simulink model "NRC_Template"  (R2025b)
settings: Solver=VariableStepAuto  StartTime=0.0  StopTime=10.0  RelTol=1e-3
undefined symbols (not defined in the file): ActivationSignal, ChargingWire, DataIN, DataLink, DataOUT, DCBus, DisplayLink, OutputWire, SwitchSignal
settings Model: Creator=jakeo  LastModifiedBy=nduka

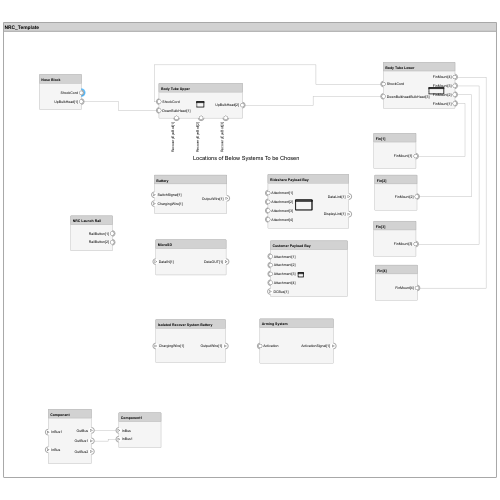
[thumbnail: Simulink's stored preview of the top-level diagram]
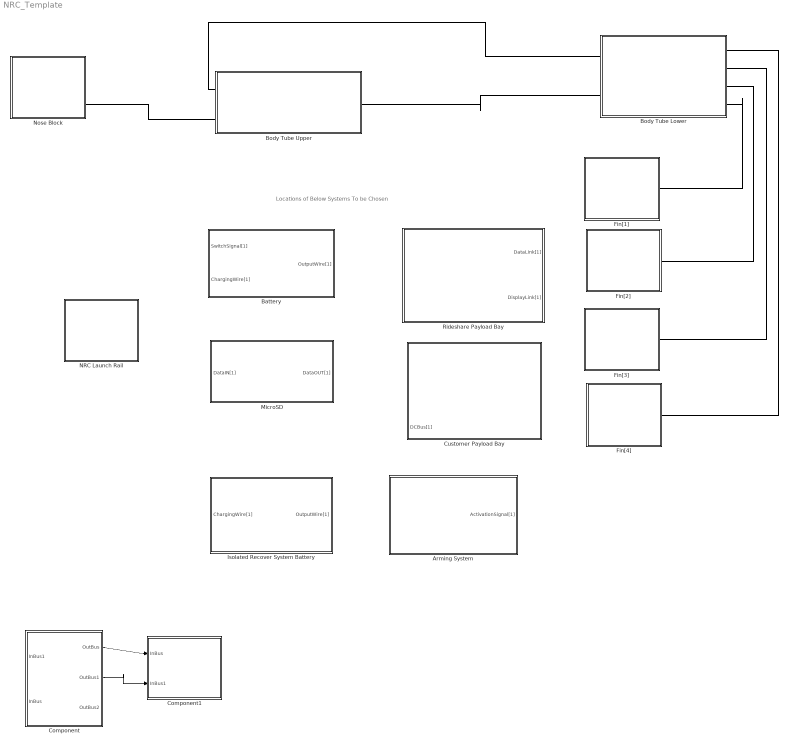
== system NRC_Template ==
  note: Locations of Below Systems To be Chosen
  Arming System : Subsystem
      settings: PortSchema="{\"entries\":[{\"content\":{\"headerSize\":26,\"margin\":15,\"minimumSpacing\":25,\"sides\":[{\"content\":{\"connectorIds\":[\"LConn1\"]},\"type\":\"ConnectorPlacement.EquallySpacedRectSide\",\"uuid\":\"6f4db608-f49c-4d1a-85cc-b66ec62c2f96\"},{\"content\":{\"connectorIds\":[\"Out1\"],\"side\":\"RIGHT\"},\"type\":\"ConnectorPlacement.EquallySpacedRectSide\",\"uuid\":\"3e275c67-1c5c-46cd-973f-75adcfca9e5d\"},{\"content\":{\"side\":\"TOP\"},\"type\":\"ConnectorPlacement.EquallySpacedRectSide\",\"uuid\":\"88fdcd36-c2bf-423f-a1bd-8e2b1c2ac438\"}]},\"type\":\"ConnectorPlacement.EquallySpacedConnector\",\"uuid\":\"596a3d77-8add-49e5-be48-e23e6a2b115a\"}],\"packageUris\":[\"http://schema.mathworks.com/mf0/Connector/R2020b\"],\"version\":\"1.0\"}"
  Battery : Subsystem
      settings: PortSchema="{\"entries\":[{\"content\":{\"headerSize\":26,\"margin\":15,\"minimumSpacing\":25,\"sides\":[{\"content\":{\"connectorIds\":[\"In1\",\"In2\"]},\"type\":\"ConnectorPlacement.EquallySpacedRectSide\",\"uuid\":\"03e957df-4bae-46ab-9d0d-48f80a496ac5\"},{\"content\":{\"connectorIds\":[\"Out1\"],\"side\":\"RIGHT\"},\"type\":\"ConnectorPlacement.EquallySpacedRectSide\",\"uuid\":\"d2433d43-ba0e-4345-8a8e-99b57dcef125\"},{\"content\":{\"side\":\"TOP\"},\"type\":\"ConnectorPlacement.EquallySpacedRectSide\",\"uuid\":\"84844adf-0e3d-439c-a28c-7cf27e8d243a\"}]},\"type\":\"ConnectorPlacement.EquallySpacedConnector\",\"uuid\":\"9b26577b-50b2-4983-8f3c-4df87f23ba49\"}],\"packageUris\":[\"http://schema.mathworks.com/mf0/Connector/R2020b\"],\"version\":\"1.0\"}"
  Body Tube Lower : Subsystem
      settings: PortSchema="{\"entries\":[{\"content\":{\"headerSize\":26,\"margin\":15,\"minimumSpacing\":25,\"sides\":[{\"content\":{\"connectorIds\":[\"LConn1\",\"LConn2\"]},\"type\":\"ConnectorPlacement.EquallySpacedRectSide\",\"uuid\":\"03e957df-4bae-46ab-9d0d-48f80a496ac5\"},{\"content\":{\"connectorIds\":[\"RConn1\",\"RConn2\",\"RConn3\",\"RConn4\"],\"side\":\"RIGHT\"},\"type\":\"ConnectorPlacement.EquallySpacedRectSide\",\"uuid\":\"d2433d43-ba0e-4345-8a8e-99b57dcef125\"},{\"content\":{\"side\":\"TOP\"},\"type\":\"ConnectorPlacement.EquallySpacedRectSide\",\"uuid\":\"84844adf-0e3d-439c-a28c-7cf27e8d243a\"}]},\"type\":\"ConnectorPlacement.EquallySpacedConnector\",\"uuid\":\"9b26577b-50b2-4983-8f3c-4df87f23ba49\"}],\"packageUris\":[\"http://schema.mathworks.com/mf0/Connector/R2020b\"],\"version\":\"1.0\"}"
  Body Tube Upper : Subsystem
      settings: PortSchema="{\"entries\":[{\"content\":{\"headerSize\":26,\"margin\":15,\"minimumSpacing\":25,\"sides\":[{\"content\":{\"connectorIds\":[\"LConn1\",\"LConn2\"]},\"type\":\"ConnectorPlacement.EquallySpacedRectSide\",\"uuid\":\"03e957df-4bae-46ab-9d0d-48f80a496ac5\"},{\"content\":{\"connectorIds\":[\"RConn1\"],\"side\":\"RIGHT\"},\"type\":\"ConnectorPlacement.EquallySpacedRectSide\",\"uuid\":\"d2433d43-ba0e-4345-8a8e-99b57dcef125\"},{\"content\":{\"side\":\"TOP\"},\"type\":\"ConnectorPlacement.EquallySpacedRectSide\",\"uuid\":\"84844adf-0e3d-439c-a28c-7cf27e8d243a\"},{\"content\":{\"connectorIds\":[\"RConn2\",\"RConn3\",\"RConn4\"],\"side\":\"BOTTOM\"},\"type\":\"ConnectorPlacement.EquallySpacedRectSide\",\"uuid\":\"7d79bddd-aaf5-48a9-85da-385393746c36\"}]},\"type\":\"ConnectorPlacement.EquallySpacedConnector\",\"uuid\":\"9b26577b-50b2-4983-8f3c-4df87f23ba49\"}],\"packageUris\":[\"http://schema.mathworks.com/mf0/Connector/R2020b\"],\"version\":\"1.0\"}"
  Component : Subsystem
      settings: PortSchema="{\"entries\":[{\"content\":{\"headerSize\":26,\"margin\":15,\"minimumSpacing\":25,\"sides\":[{\"content\":{\"connectorIds\":[\"In1\",\"In2\"]},\"type\":\"ConnectorPlacement.EquallySpacedRectSide\",\"uuid\":\"b214e6ac-d39e-436f-8c97-5d964e87c4ff\"},{\"content\":{\"connectorIds\":[\"Out1\",\"Out2\",\"Out3\"],\"side\":\"RIGHT\"},\"type\":\"ConnectorPlacement.EquallySpacedRectSide\",\"uuid\":\"c10b975c-0247-4c8e-aa32-d3b686cef9df\"},{\"content\":{\"side\":\"TOP\"},\"type\":\"ConnectorPlacement.EquallySpacedRectSide\",\"uuid\":\"84ce1942-2877-48a9-8a47-7e804e062fc7\"}]},\"type\":\"ConnectorPlacement.EquallySpacedConnector\",\"uuid\":\"8aac1783-a5cb-441e-81d2-9de359684d1e\"}],\"packageUris\":[\"http://schema.mathworks.com/mf0/Connector/R2020b\"],\"version\":\"1.0\"}"
  Component1 : Subsystem
      settings: PortSchema="{\"entries\":[{\"content\":{\"headerSize\":26,\"margin\":15,\"minimumSpacing\":25,\"sides\":[{\"content\":{\"connectorIds\":[\"In1\",\"In2\"]},\"type\":\"ConnectorPlacement.EquallySpacedRectSide\",\"uuid\":\"b214e6ac-d39e-436f-8c97-5d964e87c4ff\"},{\"content\":{\"side\":\"RIGHT\"},\"type\":\"ConnectorPlacement.EquallySpacedRectSide\",\"uuid\":\"c10b975c-0247-4c8e-aa32-d3b686cef9df\"},{\"content\":{\"side\":\"TOP\"},\"type\":\"ConnectorPlacement.EquallySpacedRectSide\",\"uuid\":\"84ce1942-2877-48a9-8a47-7e804e062fc7\"}]},\"type\":\"ConnectorPlacement.EquallySpacedConnector\",\"uuid\":\"8aac1783-a5cb-441e-81d2-9de359684d1e\"}],\"packageUris\":[\"http://schema.mathworks.com/mf0/Connector/R2020b\"],\"version\":\"1.0\"}"
  Customer Payload Bay : Subsystem
      settings: PortSchema="{\"entries\":[{\"content\":{\"headerSize\":26,\"margin\":15,\"minimumSpacing\":25,\"sides\":[{\"content\":{\"connectorIds\":[\"LConn1\",\"LConn2\",\"LConn3\",\"LConn4\",\"In1\"]},\"type\":\"ConnectorPlacement.EquallySpacedRectSide\",\"uuid\":\"03e957df-4bae-46ab-9d0d-48f80a496ac5\"},{\"content\":{\"side\":\"RIGHT\"},\"type\":\"ConnectorPlacement.EquallySpacedRectSide\",\"uuid\":\"d2433d43-ba0e-4345-8a8e-99b57dcef125\"},{\"content\":{\"side\":\"TOP\"},\"type\":\"ConnectorPlacement.EquallySpacedRectSide\",\"uuid\":\"84844adf-0e3d-439c-a28c-7cf27e8d243a\"}]},\"type\":\"ConnectorPlacement.EquallySpacedConnector\",\"uuid\":\"9b26577b-50b2-4983-8f3c-4df87f23ba49\"}],\"packageUris\":[\"http://schema.mathworks.com/mf0/Connector/R2020b\"],\"version\":\"1.0\"}"
  Fin[1] : Subsystem
      settings: PortSchema="{\"entries\":[{\"content\":{\"headerSize\":26,\"margin\":15,\"minimumSpacing\":25,\"sides\":[{\"content\":{},\"type\":\"ConnectorPlacement.EquallySpacedRectSide\",\"uuid\":\"03e957df-4bae-46ab-9d0d-48f80a496ac5\"},{\"content\":{\"connectorIds\":[\"LConn1\"],\"side\":\"RIGHT\"},\"type\":\"ConnectorPlacement.EquallySpacedRectSide\",\"uuid\":\"d2433d43-ba0e-4345-8a8e-99b57dcef125\"},{\"content\":{\"side\":\"TOP\"},\"type\":\"ConnectorPlacement.EquallySpacedRectSide\",\"uuid\":\"84844adf-0e3d-439c-a28c-7cf27e8d243a\"}]},\"type\":\"ConnectorPlacement.EquallySpacedConnector\",\"uuid\":\"9b26577b-50b2-4983-8f3c-4df87f23ba49\"}],\"packageUris\":[\"http://schema.mathworks.com/mf0/Connector/R2020b\"],\"version\":\"1.0\"}"
  Fin[2] : Subsystem
      settings: PortSchema="{\"entries\":[{\"content\":{\"headerSize\":26,\"margin\":15,\"minimumSpacing\":25,\"sides\":[{\"content\":{},\"type\":\"ConnectorPlacement.EquallySpacedRectSide\",\"uuid\":\"03e957df-4bae-46ab-9d0d-48f80a496ac5\"},{\"content\":{\"connectorIds\":[\"LConn1\"],\"side\":\"RIGHT\"},\"type\":\"ConnectorPlacement.EquallySpacedRectSide\",\"uuid\":\"d2433d43-ba0e-4345-8a8e-99b57dcef125\"},{\"content\":{\"side\":\"TOP\"},\"type\":\"ConnectorPlacement.EquallySpacedRectSide\",\"uuid\":\"84844adf-0e3d-439c-a28c-7cf27e8d243a\"}]},\"type\":\"ConnectorPlacement.EquallySpacedConnector\",\"uuid\":\"9b26577b-50b2-4983-8f3c-4df87f23ba49\"}],\"packageUris\":[\"http://schema.mathworks.com/mf0/Connector/R2020b\"],\"version\":\"1.0\"}"
  Fin[3] : Subsystem
      settings: PortSchema="{\"entries\":[{\"content\":{\"headerSize\":26,\"margin\":15,\"minimumSpacing\":25,\"sides\":[{\"content\":{},\"type\":\"ConnectorPlacement.EquallySpacedRectSide\",\"uuid\":\"03e957df-4bae-46ab-9d0d-48f80a496ac5\"},{\"content\":{\"connectorIds\":[\"LConn1\"],\"side\":\"RIGHT\"},\"type\":\"ConnectorPlacement.EquallySpacedRectSide\",\"uuid\":\"d2433d43-ba0e-4345-8a8e-99b57dcef125\"},{\"content\":{\"side\":\"TOP\"},\"type\":\"ConnectorPlacement.EquallySpacedRectSide\",\"uuid\":\"84844adf-0e3d-439c-a28c-7cf27e8d243a\"}]},\"type\":\"ConnectorPlacement.EquallySpacedConnector\",\"uuid\":\"9b26577b-50b2-4983-8f3c-4df87f23ba49\"}],\"packageUris\":[\"http://schema.mathworks.com/mf0/Connector/R2020b\"],\"version\":\"1.0\"}"
  Fin[4] : Subsystem
      settings: PortSchema="{\"entries\":[{\"content\":{\"headerSize\":26,\"margin\":15,\"minimumSpacing\":25,\"sides\":[{\"content\":{},\"type\":\"ConnectorPlacement.EquallySpacedRectSide\",\"uuid\":\"e0f0c527-1390-4ada-af2c-f34491326cf6\"},{\"content\":{\"connectorIds\":[\"RConn1\"],\"side\":\"RIGHT\"},\"type\":\"ConnectorPlacement.EquallySpacedRectSide\",\"uuid\":\"2406eba0-251b-4451-893e-81bd82ed693a\"},{\"content\":{\"side\":\"TOP\"},\"type\":\"ConnectorPlacement.EquallySpacedRectSide\",\"uuid\":\"fc9bf400-e6d0-4ec9-959a-aa9f7cd34aab\"}]},\"type\":\"ConnectorPlacement.EquallySpacedConnector\",\"uuid\":\"e5acffc5-0f25-4bd9-8a66-93873ab8fe21\"}],\"packageUris\":[\"http://schema.mathworks.com/mf0/Connector/R2020b\"],\"version\":\"1.0\"}"
  Isolated Recover System Battery : Subsystem
      settings: PortSchema="{\"entries\":[{\"content\":{\"headerSize\":26,\"margin\":15,\"minimumSpacing\":25,\"sides\":[{\"content\":{\"connectorIds\":[\"In1\"]},\"type\":\"ConnectorPlacement.EquallySpacedRectSide\",\"uuid\":\"6f4db608-f49c-4d1a-85cc-b66ec62c2f96\"},{\"content\":{\"connectorIds\":[\"Out1\"],\"side\":\"RIGHT\"},\"type\":\"ConnectorPlacement.EquallySpacedRectSide\",\"uuid\":\"3e275c67-1c5c-46cd-973f-75adcfca9e5d\"},{\"content\":{\"side\":\"TOP\"},\"type\":\"ConnectorPlacement.EquallySpacedRectSide\",\"uuid\":\"88fdcd36-c2bf-423f-a1bd-8e2b1c2ac438\"}]},\"type\":\"ConnectorPlacement.EquallySpacedConnector\",\"uuid\":\"596a3d77-8add-49e5-be48-e23e6a2b115a\"}],\"packageUris\":[\"http://schema.mathworks.com/mf0/Connector/R2020b\"],\"version\":\"1.0\"}"
  MicroSD : Subsystem
      settings: PortSchema="{\"entries\":[{\"content\":{\"headerSize\":26,\"margin\":15,\"minimumSpacing\":25,\"sides\":[{\"content\":{\"connectorIds\":[\"In1\"]},\"type\":\"ConnectorPlacement.EquallySpacedRectSide\",\"uuid\":\"6f4db608-f49c-4d1a-85cc-b66ec62c2f96\"},{\"content\":{\"connectorIds\":[\"Out1\"],\"side\":\"RIGHT\"},\"type\":\"ConnectorPlacement.EquallySpacedRectSide\",\"uuid\":\"3e275c67-1c5c-46cd-973f-75adcfca9e5d\"},{\"content\":{\"side\":\"TOP\"},\"type\":\"ConnectorPlacement.EquallySpacedRectSide\",\"uuid\":\"88fdcd36-c2bf-423f-a1bd-8e2b1c2ac438\"}]},\"type\":\"ConnectorPlacement.EquallySpacedConnector\",\"uuid\":\"596a3d77-8add-49e5-be48-e23e6a2b115a\"}],\"packageUris\":[\"http://schema.mathworks.com/mf0/Connector/R2020b\"],\"version\":\"1.0\"}"
  NRC Launch Rail : Subsystem
      settings: PortSchema="{\"entries\":[{\"content\":{\"headerSize\":26,\"margin\":15,\"minimumSpacing\":25,\"sides\":[{\"content\":{},\"type\":\"ConnectorPlacement.EquallySpacedRectSide\",\"uuid\":\"6f4db608-f49c-4d1a-85cc-b66ec62c2f96\"},{\"content\":{\"connectorIds\":[\"RConn1\",\"RConn2\"],\"side\":\"RIGHT\"},\"type\":\"ConnectorPlacement.EquallySpacedRectSide\",\"uuid\":\"3e275c67-1c5c-46cd-973f-75adcfca9e5d\"},{\"content\":{\"side\":\"TOP\"},\"type\":\"ConnectorPlacement.EquallySpacedRectSide\",\"uuid\":\"88fdcd36-c2bf-423f-a1bd-8e2b1c2ac438\"}]},\"type\":\"ConnectorPlacement.EquallySpacedConnector\",\"uuid\":\"596a3d77-8add-49e5-be48-e23e6a2b115a\"}],\"packageUris\":[\"http://schema.mathworks.com/mf0/Connector/R2020b\"],\"version\":\"1.0\"}"
  Nose Block : Subsystem
      settings: PortSchema="{\"entries\":[{\"content\":{\"headerSize\":26,\"margin\":15,\"minimumSpacing\":25,\"sides\":[{\"content\":{},\"type\":\"ConnectorPlacement.EquallySpacedRectSide\",\"uuid\":\"03e957df-4bae-46ab-9d0d-48f80a496ac5\"},{\"content\":{\"connectorIds\":[\"LConn1\",\"RConn1\"],\"side\":\"RIGHT\"},\"type\":\"ConnectorPlacement.EquallySpacedRectSide\",\"uuid\":\"d2433d43-ba0e-4345-8a8e-99b57dcef125\"},{\"content\":{\"side\":\"TOP\"},\"type\":\"ConnectorPlacement.EquallySpacedRectSide\",\"uuid\":\"84844adf-0e3d-439c-a28c-7cf27e8d243a\"}]},\"type\":\"ConnectorPlacement.EquallySpacedConnector\",\"uuid\":\"9b26577b-50b2-4983-8f3c-4df87f23ba49\"}],\"packageUris\":[\"http://schema.mathworks.com/mf0/Connector/R2020b\"],\"version\":\"1.0\"}"
  Rideshare Payload Bay : Subsystem
      settings: PortSchema="{\"entries\":[{\"content\":{\"headerSize\":26,\"margin\":15,\"minimumSpacing\":25,\"sides\":[{\"content\":{\"connectorIds\":[\"LConn1\",\"LConn2\",\"LConn3\",\"LConn4\"]},\"type\":\"ConnectorPlacement.EquallySpacedRectSide\",\"uuid\":\"03e957df-4bae-46ab-9d0d-48f80a496ac5\"},{\"content\":{\"connectorIds\":[\"Out1\",\"Out2\"],\"side\":\"RIGHT\"},\"type\":\"ConnectorPlacement.EquallySpacedRectSide\",\"uuid\":\"d2433d43-ba0e-4345-8a8e-99b57dcef125\"},{\"content\":{\"side\":\"TOP\"},\"type\":\"ConnectorPlacement.EquallySpacedRectSide\",\"uuid\":\"84844adf-0e3d-439c-a28c-7cf27e8d243a\"}]},\"type\":\"ConnectorPlacement.EquallySpacedConnector\",\"uuid\":\"9b26577b-50b2-4983-8f3c-4df87f23ba49\"}],\"packageUris\":[\"http://schema.mathworks.com/mf0/Connector/R2020b\"],\"version\":\"1.0\"}"
  wires:
  Component/1(OutBus) -> Component1/1(InBus)
  Component/2(OutBus1) -> Component1/2(InBus1)
  connections:
  Body Tube Lower/LConn1 -- Body Tube Upper/LConn1
  Nose Block/RConn1 -- Body Tube Upper/LConn2
  Body Tube Lower/LConn2 -- Body Tube Upper/RConn1
  Fin[1]/LConn1 -- Body Tube Lower/RConn4
  Fin[2]/LConn1 -- Body Tube Lower/RConn3
  Fin[3]/LConn1 -- Body Tube Lower/RConn2
  Fin[4]/RConn1 -- Body Tube Lower/RConn1

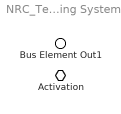
== system NRC_Template/Arming System ==
  Activation : PMIOPort  Side=Left
  Bus Element Out1 : Outport  PortName=ActivationSignal[1]

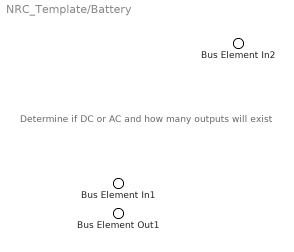
== system NRC_Template/Battery ==
  note: Determine if DC or AC and how many outputs will exist
  Bus Element In2 : Inport  PortName=SwitchSignal[1]
  Bus Element In1 : Inport  Port=2  PortName=ChargingWire[1]
  Bus Element Out1 : Outport  PortName=OutputWire[1]

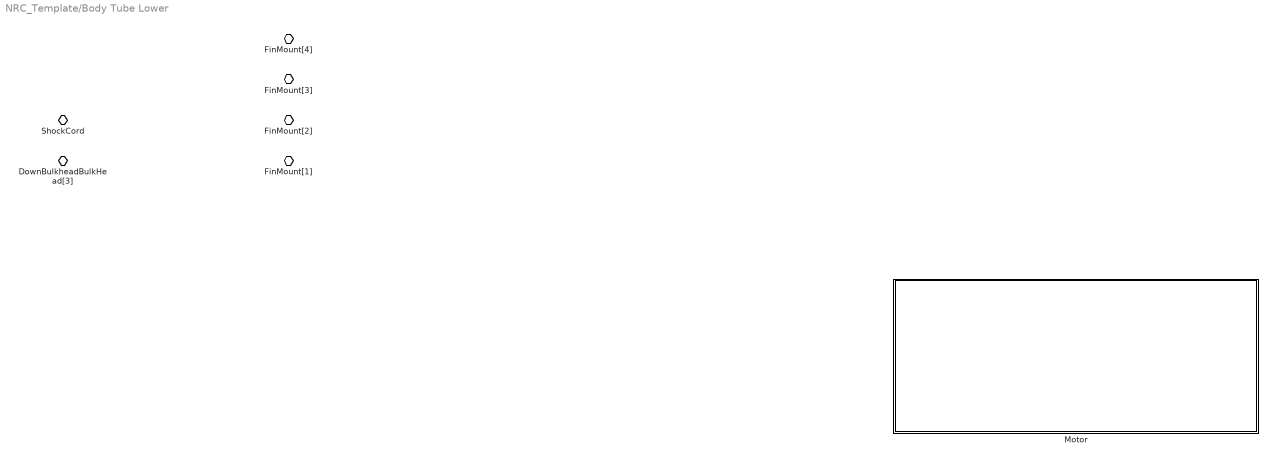
== system NRC_Template/Body Tube Lower ==
  Motor : Subsystem
      settings: PortSchema="{\"entries\":[{\"content\":{\"headerSize\":26,\"margin\":15,\"minimumSpacing\":25,\"sides\":[{\"content\":{\"connectorIds\":[\"LConn1\",\"LConn2\"]},\"type\":\"ConnectorPlacement.EquallySpacedRectSide\",\"uuid\":\"03e957df-4bae-46ab-9d0d-48f80a496ac5\"},{\"content\":{\"side\":\"RIGHT\"},\"type\":\"ConnectorPlacement.EquallySpacedRectSide\",\"uuid\":\"d2433d43-ba0e-4345-8a8e-99b57dcef125\"},{\"content\":{\"side\":\"TOP\"},\"type\":\"ConnectorPlacement.EquallySpacedRectSide\",\"uuid\":\"84844adf-0e3d-439c-a28c-7cf27e8d243a\"}]},\"type\":\"ConnectorPlacement.EquallySpacedConnector\",\"uuid\":\"9b26577b-50b2-4983-8f3c-4df87f23ba49\"}],\"packageUris\":[\"http://schema.mathworks.com/mf0/Connector/R2020b\"],\"version\":\"1.0\"}"
  ShockCord : PMIOPort  Side=Left
  DownBulkheadBulkHead[3] : PMIOPort  Port=2  Side=Left
  FinMount[4] : PMIOPort  Port=3  Side=Right
  FinMount[3] : PMIOPort  Port=4  Side=Right
  FinMount[2] : PMIOPort  Port=5  Side=Right
  FinMount[1] : PMIOPort  Port=6  Side=Right

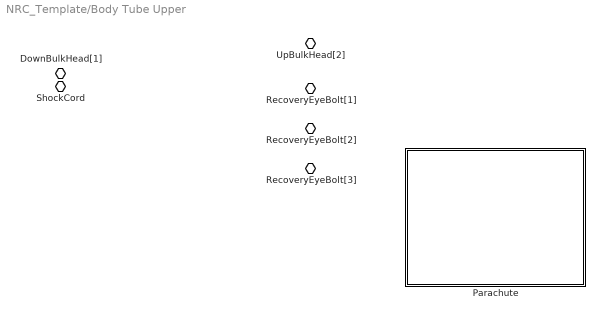
== system NRC_Template/Body Tube Upper ==
  Parachute : Subsystem
      settings: PortSchema="{\"entries\":[{\"content\":{\"headerSize\":26,\"margin\":15,\"minimumSpacing\":25,\"sides\":[{\"content\":{\"connectorIds\":[\"LConn1\",\"LConn2\",\"LConn3\"]},\"type\":\"ConnectorPlacement.EquallySpacedRectSide\",\"uuid\":\"03e957df-4bae-46ab-9d0d-48f80a496ac5\"},{\"content\":{\"side\":\"RIGHT\"},\"type\":\"ConnectorPlacement.EquallySpacedRectSide\",\"uuid\":\"d2433d43-ba0e-4345-8a8e-99b57dcef125\"},{\"content\":{\"side\":\"TOP\"},\"type\":\"ConnectorPlacement.EquallySpacedRectSide\",\"uuid\":\"84844adf-0e3d-439c-a28c-7cf27e8d243a\"}]},\"type\":\"ConnectorPlacement.EquallySpacedConnector\",\"uuid\":\"9b26577b-50b2-4983-8f3c-4df87f23ba49\"}],\"packageUris\":[\"http://schema.mathworks.com/mf0/Connector/R2020b\"],\"version\":\"1.0\"}"
  ShockCord : PMIOPort  Side=Left
  DownBulkHead[1] : PMIOPort  Port=2  Side=Left
  UpBulkHead[2] : PMIOPort  Port=3  Side=Right
  RecoveryEyeBolt[1] : PMIOPort  Port=4  Side=Right
  RecoveryEyeBolt[2] : PMIOPort  Port=5  Side=Right
  RecoveryEyeBolt[3] : PMIOPort  Port=6  Side=Right

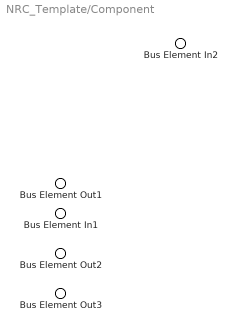
== system NRC_Template/Component ==
  Bus Element In2 : Inport  PortName=InBus1
  Bus Element In1 : Inport  Port=2  PortName=InBus
  Bus Element Out1 : Outport  PortName=OutBus
  Bus Element Out2 : Outport  Port=2  PortName=OutBus1
  Bus Element Out3 : Outport  Port=3  PortName=OutBus2

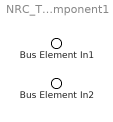
== system NRC_Template/Component1 ==
  Bus Element In1 : Inport  PortName=InBus
  Bus Element In2 : Inport  Port=2  PortName=InBus1

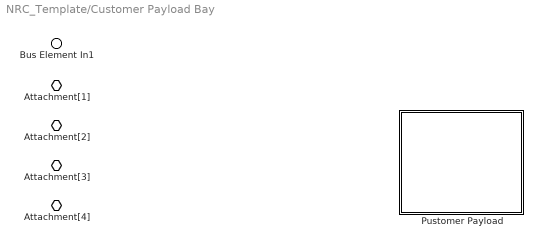
== system NRC_Template/Customer Payload Bay ==
  Bus Element In1 : Inport  PortName=DCBus[1]
  Pustomer Payload : Subsystem
      settings: PortSchema="{\"entries\":[{\"content\":{\"headerSize\":26,\"margin\":15,\"minimumSpacing\":25,\"sides\":[{\"content\":{\"connectorIds\":[\"LConn1\"]},\"type\":\"ConnectorPlacement.EquallySpacedRectSide\",\"uuid\":\"03e957df-4bae-46ab-9d0d-48f80a496ac5\"},{\"content\":{\"side\":\"RIGHT\"},\"type\":\"ConnectorPlacement.EquallySpacedRectSide\",\"uuid\":\"d2433d43-ba0e-4345-8a8e-99b57dcef125\"},{\"content\":{\"side\":\"TOP\"},\"type\":\"ConnectorPlacement.EquallySpacedRectSide\",\"uuid\":\"84844adf-0e3d-439c-a28c-7cf27e8d243a\"}]},\"type\":\"ConnectorPlacement.EquallySpacedConnector\",\"uuid\":\"9b26577b-50b2-4983-8f3c-4df87f23ba49\"}],\"packageUris\":[\"http://schema.mathworks.com/mf0/Connector/R2020b\"],\"version\":\"1.0\"}"
  Attachment[1] : PMIOPort  Side=Left
  Attachment[2] : PMIOPort  Port=2  Side=Left
  Attachment[3] : PMIOPort  Port=3  Side=Left
  Attachment[4] : PMIOPort  Port=4  Side=Left

== system NRC_Template/Fin[1] ==
  FinMount[1] : PMIOPort  Side=Left

== system NRC_Template/Fin[2] ==
  FinMount[2] : PMIOPort  Side=Left

== system NRC_Template/Fin[3] ==
  FinMount[3] : PMIOPort  Side=Left

== system NRC_Template/Fin[4] ==
  FinMount[4] : PMIOPort  Side=Right

== system NRC_Template/Isolated Recover System Battery ==
  Bus Element In1 : Inport  PortName=ChargingWire[1]
  Bus Element Out1 : Outport  PortName=OutputWire[1]

== system NRC_Template/MicroSD ==
  Bus Element In1 : Inport  PortName=DataIN[1]
  Bus Element Out1 : Outport  PortName=DataOUT[1]

== system NRC_Template/NRC Launch Rail ==
  RailButton[1] : PMIOPort  Side=Right
  RailButton[2] : PMIOPort  Port=2  Side=Right

== system NRC_Template/Nose Block ==
  ShockCord : PMIOPort  Side=Left
  UpBulkHead[1] : PMIOPort  Port=2  Side=Right

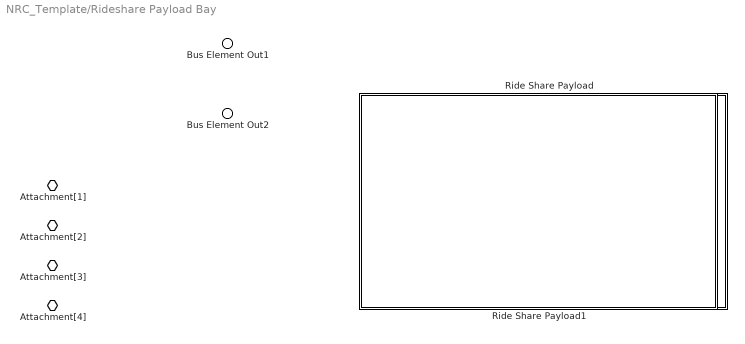
== system NRC_Template/Rideshare Payload Bay ==
  Ride Share Payload : Subsystem
      settings: PortSchema="{\"entries\":[{\"content\":{\"headerSize\":26,\"margin\":15,\"minimumSpacing\":25,\"sides\":[{\"content\":{},\"type\":\"ConnectorPlacement.EquallySpacedRectSide\",\"uuid\":\"03e957df-4bae-46ab-9d0d-48f80a496ac5\"},{\"content\":{\"side\":\"RIGHT\"},\"type\":\"ConnectorPlacement.EquallySpacedRectSide\",\"uuid\":\"d2433d43-ba0e-4345-8a8e-99b57dcef125\"},{\"content\":{\"side\":\"TOP\"},\"type\":\"ConnectorPlacement.EquallySpacedRectSide\",\"uuid\":\"84844adf-0e3d-439c-a28c-7cf27e8d243a\"}]},\"type\":\"ConnectorPlacement.EquallySpacedConnector\",\"uuid\":\"9b26577b-50b2-4983-8f3c-4df87f23ba49\"}],\"packageUris\":[\"http://schema.mathworks.com/mf0/Connector/R2020b\"],\"version\":\"1.0\"}"
  Ride Share Payload1 : Subsystem
      settings: PortSchema="{\"entries\":[{\"content\":{\"headerSize\":26,\"margin\":15,\"minimumSpacing\":25,\"sides\":[{\"content\":{},\"type\":\"ConnectorPlacement.EquallySpacedRectSide\",\"uuid\":\"03e957df-4bae-46ab-9d0d-48f80a496ac5\"},{\"content\":{\"side\":\"RIGHT\"},\"type\":\"ConnectorPlacement.EquallySpacedRectSide\",\"uuid\":\"d2433d43-ba0e-4345-8a8e-99b57dcef125\"},{\"content\":{\"side\":\"TOP\"},\"type\":\"ConnectorPlacement.EquallySpacedRectSide\",\"uuid\":\"84844adf-0e3d-439c-a28c-7cf27e8d243a\"}]},\"type\":\"ConnectorPlacement.EquallySpacedConnector\",\"uuid\":\"9b26577b-50b2-4983-8f3c-4df87f23ba49\"}],\"packageUris\":[\"http://schema.mathworks.com/mf0/Connector/R2020b\"],\"version\":\"1.0\"}"
  Attachment[1] : PMIOPort  Side=Left
  Attachment[2] : PMIOPort  Port=2  Side=Left
  Attachment[3] : PMIOPort  Port=3  Side=Left
  Attachment[4] : PMIOPort  Port=4  Side=Left
  Bus Element Out1 : Outport  PortName=DataLink[1]
  Bus Element Out2 : Outport  Port=2  PortName=DisplayLink[1]

== system NRC_Template/Body Tube Lower/Motor ==
  Mount[1] : PMIOPort  Side=Left
  Mount[2] : PMIOPort  Port=2  Side=Left

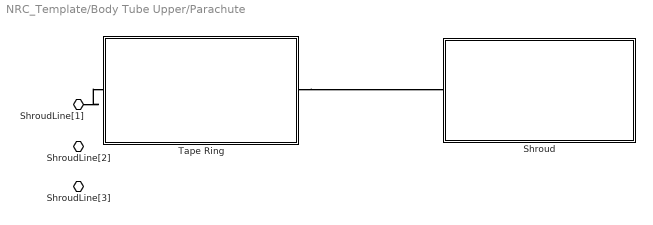
== system NRC_Template/Body Tube Upper/Parachute ==
  Shroud : Subsystem
      settings: PortSchema="{\"entries\":[{\"content\":{\"headerSize\":26,\"margin\":15,\"minimumSpacing\":25,\"sides\":[{\"content\":{\"connectorIds\":[\"LConn1\"]},\"type\":\"ConnectorPlacement.EquallySpacedRectSide\",\"uuid\":\"03e957df-4bae-46ab-9d0d-48f80a496ac5\"},{\"content\":{\"side\":\"RIGHT\"},\"type\":\"ConnectorPlacement.EquallySpacedRectSide\",\"uuid\":\"d2433d43-ba0e-4345-8a8e-99b57dcef125\"},{\"content\":{\"side\":\"TOP\"},\"type\":\"ConnectorPlacement.EquallySpacedRectSide\",\"uuid\":\"84844adf-0e3d-439c-a28c-7cf27e8d243a\"}]},\"type\":\"ConnectorPlacement.EquallySpacedConnector\",\"uuid\":\"9b26577b-50b2-4983-8f3c-4df87f23ba49\"}],\"packageUris\":[\"http://schema.mathworks.com/mf0/Connector/R2020b\"],\"version\":\"1.0\"}"
  Tape Ring : Subsystem
      settings: PortSchema="{\"entries\":[{\"content\":{\"headerSize\":26,\"margin\":15,\"minimumSpacing\":25,\"sides\":[{\"content\":{\"connectorIds\":[\"LConn1\"]},\"type\":\"ConnectorPlacement.EquallySpacedRectSide\",\"uuid\":\"03e957df-4bae-46ab-9d0d-48f80a496ac5\"},{\"content\":{\"connectorIds\":[\"RConn1\"],\"side\":\"RIGHT\"},\"type\":\"ConnectorPlacement.EquallySpacedRectSide\",\"uuid\":\"d2433d43-ba0e-4345-8a8e-99b57dcef125\"},{\"content\":{\"side\":\"TOP\"},\"type\":\"ConnectorPlacement.EquallySpacedRectSide\",\"uuid\":\"84844adf-0e3d-439c-a28c-7cf27e8d243a\"}]},\"type\":\"ConnectorPlacement.EquallySpacedConnector\",\"uuid\":\"9b26577b-50b2-4983-8f3c-4df87f23ba49\"}],\"packageUris\":[\"http://schema.mathworks.com/mf0/Connector/R2020b\"],\"version\":\"1.0\"}"
  ShroudLine[1] : PMIOPort  Side=Left
  ShroudLine[2] : PMIOPort  Port=2  Side=Left
  ShroudLine[3] : PMIOPort  Port=3  Side=Left
  connections:
  ShroudLine[1]/RConn1 -- Tape Ring/LConn1
  Tape Ring/RConn1 -- Shroud/LConn1

== system NRC_Template/Customer Payload Bay/Pustomer Payload ==
  DCBus[1] : PMIOPort  Side=Left

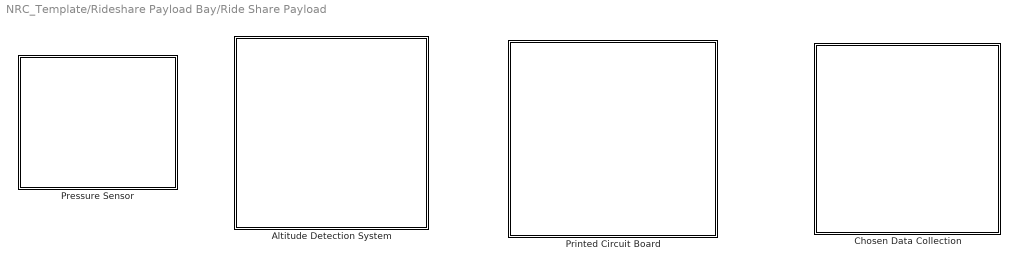
== system NRC_Template/Rideshare Payload Bay/Ride Share Payload ==
  Altitude Detection System : Subsystem
      settings: PortSchema="{\"entries\":[{\"content\":{\"headerSize\":26,\"margin\":15,\"minimumSpacing\":25,\"sides\":[{\"content\":{},\"type\":\"ConnectorPlacement.EquallySpacedRectSide\",\"uuid\":\"6f4db608-f49c-4d1a-85cc-b66ec62c2f96\"},{\"content\":{\"side\":\"RIGHT\"},\"type\":\"ConnectorPlacement.EquallySpacedRectSide\",\"uuid\":\"3e275c67-1c5c-46cd-973f-75adcfca9e5d\"},{\"content\":{\"side\":\"TOP\"},\"type\":\"ConnectorPlacement.EquallySpacedRectSide\",\"uuid\":\"88fdcd36-c2bf-423f-a1bd-8e2b1c2ac438\"}]},\"type\":\"ConnectorPlacement.EquallySpacedConnector\",\"uuid\":\"596a3d77-8add-49e5-be48-e23e6a2b115a\"}],\"packageUris\":[\"http://schema.mathworks.com/mf0/Connector/R2020b\"],\"version\":\"1.0\"}"
  Chosen Data Collection : Subsystem
      settings: PortSchema="{\"entries\":[{\"content\":{\"headerSize\":26,\"margin\":15,\"minimumSpacing\":25,\"sides\":[{\"content\":{},\"type\":\"ConnectorPlacement.EquallySpacedRectSide\",\"uuid\":\"6f4db608-f49c-4d1a-85cc-b66ec62c2f96\"},{\"content\":{\"side\":\"RIGHT\"},\"type\":\"ConnectorPlacement.EquallySpacedRectSide\",\"uuid\":\"3e275c67-1c5c-46cd-973f-75adcfca9e5d\"},{\"content\":{\"side\":\"TOP\"},\"type\":\"ConnectorPlacement.EquallySpacedRectSide\",\"uuid\":\"88fdcd36-c2bf-423f-a1bd-8e2b1c2ac438\"}]},\"type\":\"ConnectorPlacement.EquallySpacedConnector\",\"uuid\":\"596a3d77-8add-49e5-be48-e23e6a2b115a\"}],\"packageUris\":[\"http://schema.mathworks.com/mf0/Connector/R2020b\"],\"version\":\"1.0\"}"
  "Pressure Sensor " : Subsystem
      settings: PortSchema="{\"entries\":[{\"content\":{\"headerSize\":26,\"margin\":15,\"minimumSpacing\":25,\"sides\":[{\"content\":{},\"type\":\"ConnectorPlacement.EquallySpacedRectSide\",\"uuid\":\"1f2b9a1d-6713-4d6c-9fa5-a9776360dec0\"},{\"content\":{\"side\":\"RIGHT\"},\"type\":\"ConnectorPlacement.EquallySpacedRectSide\",\"uuid\":\"ac44a9c5-24d9-43ce-9c8b-ca9143b25fb3\"},{\"content\":{\"side\":\"TOP\"},\"type\":\"ConnectorPlacement.EquallySpacedRectSide\",\"uuid\":\"a5d57953-b9e9-476d-bb67-374b6d9b1c76\"}]},\"type\":\"ConnectorPlacement.EquallySpacedConnector\",\"uuid\":\"8953d32c-651c-4cfa-821f-8f95c4d18772\"}],\"packageUris\":[\"http://schema.mathworks.com/mf0/Connector/R2020b\"],\"version\":\"1.0\"}"
  Printed Circuit Board : Subsystem
      settings: PortSchema="{\"entries\":[{\"content\":{\"headerSize\":26,\"margin\":15,\"minimumSpacing\":25,\"sides\":[{\"content\":{},\"type\":\"ConnectorPlacement.EquallySpacedRectSide\",\"uuid\":\"6f4db608-f49c-4d1a-85cc-b66ec62c2f96\"},{\"content\":{\"side\":\"RIGHT\"},\"type\":\"ConnectorPlacement.EquallySpacedRectSide\",\"uuid\":\"3e275c67-1c5c-46cd-973f-75adcfca9e5d\"},{\"content\":{\"side\":\"TOP\"},\"type\":\"ConnectorPlacement.EquallySpacedRectSide\",\"uuid\":\"88fdcd36-c2bf-423f-a1bd-8e2b1c2ac438\"}]},\"type\":\"ConnectorPlacement.EquallySpacedConnector\",\"uuid\":\"596a3d77-8add-49e5-be48-e23e6a2b115a\"}],\"packageUris\":[\"http://schema.mathworks.com/mf0/Connector/R2020b\"],\"version\":\"1.0\"}"

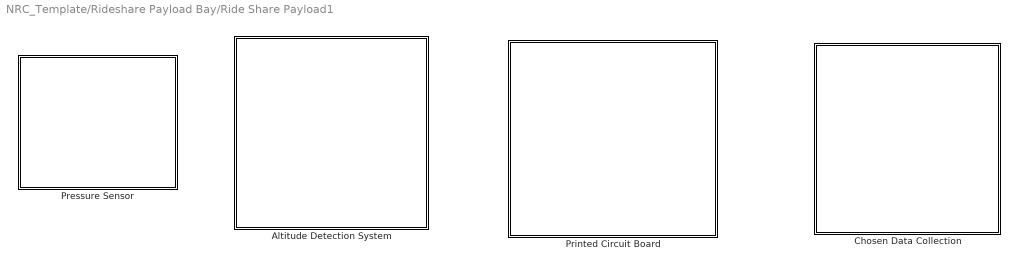
== system NRC_Template/Rideshare Payload Bay/Ride Share Payload1 ==
  Altitude Detection System : Subsystem
      settings: PortSchema="{\"entries\":[{\"content\":{\"headerSize\":26,\"margin\":15,\"minimumSpacing\":25,\"sides\":[{\"content\":{},\"type\":\"ConnectorPlacement.EquallySpacedRectSide\",\"uuid\":\"6f4db608-f49c-4d1a-85cc-b66ec62c2f96\"},{\"content\":{\"side\":\"RIGHT\"},\"type\":\"ConnectorPlacement.EquallySpacedRectSide\",\"uuid\":\"3e275c67-1c5c-46cd-973f-75adcfca9e5d\"},{\"content\":{\"side\":\"TOP\"},\"type\":\"ConnectorPlacement.EquallySpacedRectSide\",\"uuid\":\"88fdcd36-c2bf-423f-a1bd-8e2b1c2ac438\"}]},\"type\":\"ConnectorPlacement.EquallySpacedConnector\",\"uuid\":\"596a3d77-8add-49e5-be48-e23e6a2b115a\"}],\"packageUris\":[\"http://schema.mathworks.com/mf0/Connector/R2020b\"],\"version\":\"1.0\"}"
  Chosen Data Collection : Subsystem
      settings: PortSchema="{\"entries\":[{\"content\":{\"headerSize\":26,\"margin\":15,\"minimumSpacing\":25,\"sides\":[{\"content\":{},\"type\":\"ConnectorPlacement.EquallySpacedRectSide\",\"uuid\":\"6f4db608-f49c-4d1a-85cc-b66ec62c2f96\"},{\"content\":{\"side\":\"RIGHT\"},\"type\":\"ConnectorPlacement.EquallySpacedRectSide\",\"uuid\":\"3e275c67-1c5c-46cd-973f-75adcfca9e5d\"},{\"content\":{\"side\":\"TOP\"},\"type\":\"ConnectorPlacement.EquallySpacedRectSide\",\"uuid\":\"88fdcd36-c2bf-423f-a1bd-8e2b1c2ac438\"}]},\"type\":\"ConnectorPlacement.EquallySpacedConnector\",\"uuid\":\"596a3d77-8add-49e5-be48-e23e6a2b115a\"}],\"packageUris\":[\"http://schema.mathworks.com/mf0/Connector/R2020b\"],\"version\":\"1.0\"}"
  "Pressure Sensor " : Subsystem
      settings: PortSchema="{\"entries\":[{\"content\":{\"headerSize\":26,\"margin\":15,\"minimumSpacing\":25,\"sides\":[{\"content\":{},\"type\":\"ConnectorPlacement.EquallySpacedRectSide\",\"uuid\":\"1f2b9a1d-6713-4d6c-9fa5-a9776360dec0\"},{\"content\":{\"side\":\"RIGHT\"},\"type\":\"ConnectorPlacement.EquallySpacedRectSide\",\"uuid\":\"ac44a9c5-24d9-43ce-9c8b-ca9143b25fb3\"},{\"content\":{\"side\":\"TOP\"},\"type\":\"ConnectorPlacement.EquallySpacedRectSide\",\"uuid\":\"a5d57953-b9e9-476d-bb67-374b6d9b1c76\"}]},\"type\":\"ConnectorPlacement.EquallySpacedConnector\",\"uuid\":\"8953d32c-651c-4cfa-821f-8f95c4d18772\"}],\"packageUris\":[\"http://schema.mathworks.com/mf0/Connector/R2020b\"],\"version\":\"1.0\"}"
  Printed Circuit Board : Subsystem
      settings: PortSchema="{\"entries\":[{\"content\":{\"headerSize\":26,\"margin\":15,\"minimumSpacing\":25,\"sides\":[{\"content\":{},\"type\":\"ConnectorPlacement.EquallySpacedRectSide\",\"uuid\":\"6f4db608-f49c-4d1a-85cc-b66ec62c2f96\"},{\"content\":{\"side\":\"RIGHT\"},\"type\":\"ConnectorPlacement.EquallySpacedRectSide\",\"uuid\":\"3e275c67-1c5c-46cd-973f-75adcfca9e5d\"},{\"content\":{\"side\":\"TOP\"},\"type\":\"ConnectorPlacement.EquallySpacedRectSide\",\"uuid\":\"88fdcd36-c2bf-423f-a1bd-8e2b1c2ac438\"}]},\"type\":\"ConnectorPlacement.EquallySpacedConnector\",\"uuid\":\"596a3d77-8add-49e5-be48-e23e6a2b115a\"}],\"packageUris\":[\"http://schema.mathworks.com/mf0/Connector/R2020b\"],\"version\":\"1.0\"}"

== system NRC_Template/Body Tube Upper/Parachute/Shroud ==
  ShroudLines[2] : PMIOPort  Side=Left

== system NRC_Template/Body Tube Upper/Parachute/Tape Ring ==
  ShroudLines[1] : PMIOPort  Side=Left
  ShroudLines[2] : PMIOPort  Port=2  Side=Right

== system NRC_Template/Rideshare Payload Bay/Ride Share Payload/Altitude Detection System ==

== system NRC_Template/Rideshare Payload Bay/Ride Share Payload/Chosen Data Collection ==

== system NRC_Template/Rideshare Payload Bay/Ride Share Payload/Pressure Sensor  ==

== system NRC_Template/Rideshare Payload Bay/Ride Share Payload/Printed Circuit Board ==

== system NRC_Template/Rideshare Payload Bay/Ride Share Payload1/Altitude Detection System ==

== system NRC_Template/Rideshare Payload Bay/Ride Share Payload1/Chosen Data Collection ==

== system NRC_Template/Rideshare Payload Bay/Ride Share Payload1/Pressure Sensor  ==

== system NRC_Template/Rideshare Payload Bay/Ride Share Payload1/Printed Circuit Board ==
